simulink model "Mass_spring_system"  (R2023b)
settings: Solver=VariableStepAuto  StartTime=0.0  StopTime=100  MaxStep=0.01  RelTol=1e-3
settings Model: Creator=91839  LastModifiedBy=siva kumar
settings SolverCC: AlgebraicLoopSolver=TrustRegion
settings DataIOCC: ExternalInput=data  SaveFormat=Array  DSMLogging=off  ReturnWorkspaceOutputs=off
settings DebuggingCC: UnconnectedInputMsg=warning  UnconnectedOutputMsg=warning  UnconnectedLineMsg=warning
settings ModelReferenceCC: EnableRefExpFcnMdlSchedulingChecks=on
settings SFSimCC: CustomCodeUndefinedFunction=UseInterfaceOnly

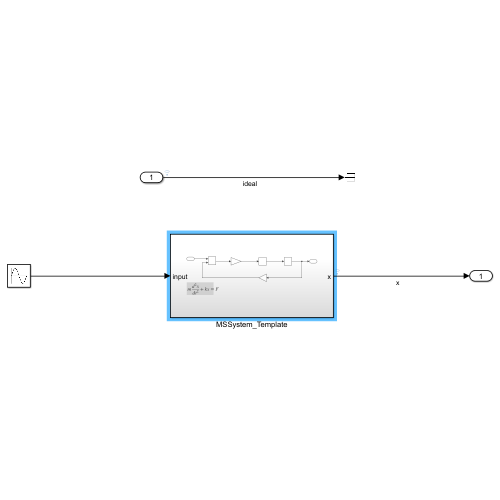
[thumbnail: Simulink's stored preview of the top-level diagram]
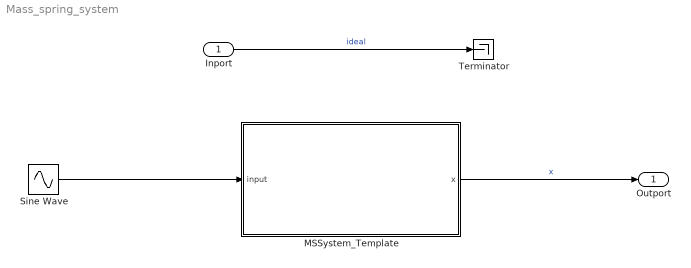
== system Mass_spring_system ==
  Inport : Inport
  MSSystem_Template : Subsystem
  Sine Wave : Sin  SampleTime=0
  Terminator : Terminator
  Outport : Outport
  wires:
  Inport/1 -> Terminator/1  "ideal"
  Sine Wave/1 -> MSSystem_Template/1(input)
  MSSystem_Template/1(x) -> Outport/1  "x"

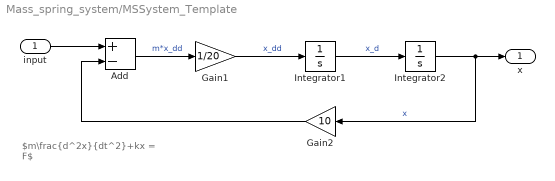
== system Mass_spring_system/MSSystem_Template ==
  note: $m\frac{d^2x}{dt^2}+kx = F$
  input : Inport
  Add : Sum  Inputs=+-
  Gain1 : Gain  Gain=1/20
  Gain2 : Gain  Gain=10
  Integrator1 : Integrator
  Integrator2 : Integrator  InitialCondition=1
  x : Outport
  wires:
  input/1 -> Add/1
  Add/1 -> Gain1/1  "m*x_dd"
  Gain1/1 -> Integrator1/1  "x_dd"
  Integrator1/1 -> Integrator2/1  "x_d"
  Integrator2/1 -> Gain2/1, x/1  "x"
  Gain2/1 -> Add/2
